simulink model "E_c_Linearizovana_staticka_karakteristika_20_80"  (R2016a)
settings: Solver=VariableStepAuto  StartTime=0.0  StopTime=800  RelTol=1e-3
libraries: simulink x2
settings Model: Creator=AmelT  LastModifiedBy=AmelT

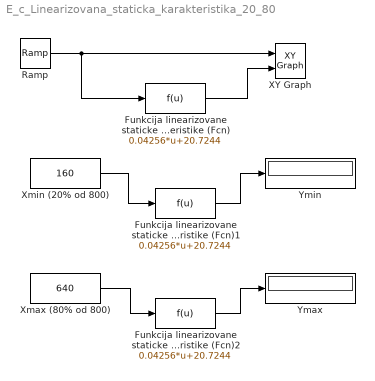
== system E_c_Linearizovana_staticka_karakteristika_20_80 ==
  Funkcija linearizovane staticke karakteristike (Fcn) : Fcn  Expr=0.04256*u+20.7244
  Funkcija linearizovane staticke karakteristike (Fcn)1 : Fcn  Expr=0.04256*u+20.7244
  Funkcija linearizovane staticke karakteristike (Fcn)2 : Fcn  Expr=0.04256*u+20.7244
  Ramp : simulink/Sources/Ramp  slope=1  start=0  X0=0
  XY Graph : simulink/Sinks/XY Graph  xmin=0  xmax=800  ymin=0  ymax=50  st=1
  Xmax (80% od 800) : Constant  Value=640
  Xmin (20% od 800) : Constant  Value=160
  Ymax : Display
  Ymin : Display
  wires:
  Ramp/1 -> Funkcija linearizovane staticke karakteristike (Fcn)/1, XY Graph/1
  Funkcija linearizovane staticke karakteristike (Fcn)/1 -> XY Graph/2
  Xmin (20% od 800)/1 -> Funkcija linearizovane staticke karakteristike (Fcn)1/1
  Funkcija linearizovane staticke karakteristike (Fcn)1/1 -> Ymin/1
  Xmax (80% od 800)/1 -> Funkcija linearizovane staticke karakteristike (Fcn)2/1
  Funkcija linearizovane staticke karakteristike (Fcn)2/1 -> Ymax/1
